simulink model "StateFlowForLoop"  (R2020a)
settings: Solver=VariableStepAuto  StartTime=0.0  StopTime=10.0  RelTol=1e-3
libraries: simulink x1
settings Model: Creator=ashok  LastModifiedBy=ashok

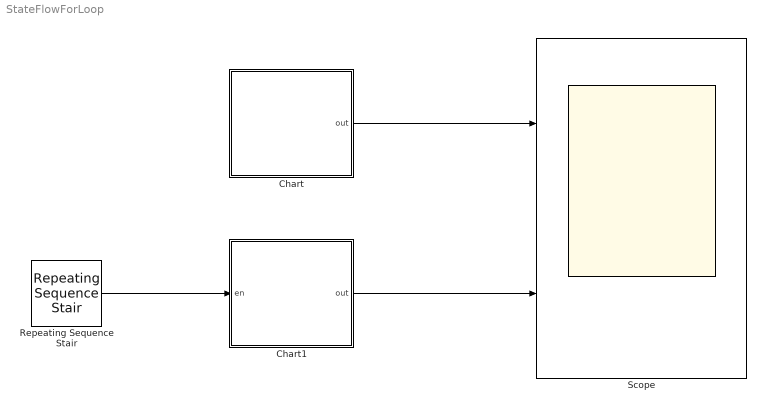
== system StateFlowForLoop ==
  Chart : Stateflow chart  TreatAsAtomicUnit=on
  Chart1 : Stateflow chart  TreatAsAtomicUnit=on
  Repeating Sequence Stair : simulink/Sources/Repeating Sequence Stair  OutValues=[0 1].'  tsamp=-1  OutMin=[]  OutMax=[]  OutDataTypeStr=double  OutputDataTypeScalingMode=double  OutDataType=fixdt(0,8)  ConRadixGroup=Best Precision: Vector-wise  OutScaling=2^-12
  Scope : Scope  NumInputPorts=2
  wires:
  Repeating Sequence Stair/1 -> Chart1/1(en)
  Chart1/1(out) -> Scope/2
  Chart/1(out) -> Scope/1

== stateflow chart StateFlowForLoop/Chart1 ==
  (default) -> (junction 14) : {i = 0;
      | out = 0;
      | }
  (junction 28) -> (junction 31) [order 1] : [i<=10]
  (junction 31) -> (junction 32) : {out = out + i;}
  (junction 14) -> (junction 28) [order 1] : [en == 1]
  (junction 32) -> (junction 28) : {i = i+1;}
  (junction 14) -> (junction 17) [order 2]
  (junction 28) -> (junction 23) [order 2]
  (junction 23) -> (junction 17)
  data: i local size=1; out output; en input

== stateflow chart StateFlowForLoop/Chart ==
  (default) -> (junction 3) : {i = 0;
      | out = 0;}
  (junction 3) -> (junction 7) [order 1] : [ i <= 10]
  (junction 7) -> (junction 8) : {out = out + i;}
  (junction 8) -> (junction 3) : { i = i+1;}
  (junction 3) -> (junction 5) [order 2]
  data: i local size=1; out output
